simulink model "FM_Tut1"  (R2021a)
settings: Solver=VariableStepAuto  StartTime=0.0  StopTime=10.0  RelTol=1e-3
model workspace (MAT data in the model file):
  Ts = 4.16666666667e-06
  kf = 75000
libraries: dsparch4 x2, dspsnks4 x1, rtlsdr_book_library x1, dspstat3 x1, sdrrlib x1
settings Model: Creator=devan  LastModifiedBy=devan

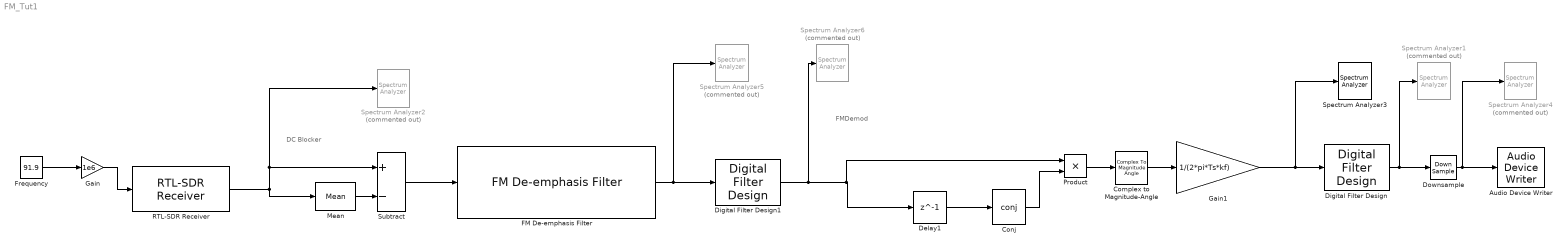
== system FM_Tut1 ==
  note: FMDemod
  note: DC Blocker
  Audio Device Writer : dspsnks4/Audio Device Writer  Driver=DirectSound  Device=Default  InheritSampleRate=on  SampleRate=44100  BitDepth=16-bit integer  BufferSize=4096  NumBuffers=10  DefaultOutputChannelMapping=on  OutputChannelMapping=1:2  OutputNumUnderrunSamples=off  DriverIdx=1  DeviceWarnFlag=''
  Complex to Magnitude-Angle : ComplexToMagnitudeAngle  Output=Angle
  Conj : Math  Operator=conj  SaturateOnIntegerOverflow=on
  Delay1 : Delay  DelayLength=1  InputProcessing=Columns as channels (frame based)
  Digital Filter Design : dsparch4/Digital Filter Design  mwdsp_browser_bugfix_var=off
  Digital Filter Design1 : dsparch4/Digital Filter Design  mwdsp_browser_bugfix_var=off
  Downsample : DownSample  N=5
  FM De-emphasis Filter : rtlsdr_book_library/FM Demod Tools/FM De-emphasis Filter  region=Europe, Asia  fs=240e3
      settings: SourceProductName=RTL-SDR Book Library
  Frequency : Constant  Value=91.9
  Gain : Gain  Gain=1e6
  Gain1 : Gain  Gain=1/(2*pi*Ts*kf)
  Mean : dspstat3/Mean  run=off  InputProcessing=Columns as channels (frame based)  reset_popup=None  directionMode=Each column  dimension=1  roiEnable=off  roiType=Rectangles  roiPortion=Entire ROI  roiOutput=Individual statistics for each ROI  roiFlag=off  roundingMode=Floor  overflowMode=off  outputDataTypeStr=Inherit: Same as accumulator  outputMin=[]  outputMax=[]  outputLastDataTypeStr=Inherit: Same as accumulator
  Product : Product
  RTL-SDR Receiver : sdrrlib/RTL-SDR Receiver  IPAddress=0  CenterFrequencySource=Input port  CenterFrequency=102.5e6  GainSource=Dialog  Gain=25  ADCRate=240e3  FrequencyCorrection=0  LostSamplesOutputPort=off  LatencyOutputPort=off  OutputDataType=single  FrameLength=1000  EnableBurstMode=off  NumFramesInBurst=20  sobjType=sdrr.internal.SDRRTLReceiverSL  dataUDPPort=-1  ctrlUDPPort=-1  subDeviceList=nosubdev  sdrBlockType=SDRBlockTypeSLT.SDRRxBlock  requester=UNUSED_BY_SFCN  sdrExecutionMode=SDRExecutionModeSLT.ExecModeHW  BypassUserLogic=off  DecimatorSelect=DDC decimator  SourceSelect=RF data  SineAmplitude=16000  EnableInternalClock=off  BypassIQBalance=off  IFBandwidth=40e6  ADCRateSource=Dialog  IntermediateFrequency=0  DecimationFactorSource=Dialog  DecimationFactor=512  RFFrequencyIsTunable=logical(1)  SampleTime=(1000)/(240e3)  IFBandwidthSource=Dialog  SineFrequency=30000  BypassDCBlockingFilter=off  IntermediateFrequencySource=Dialog  IQBalanceCoefficients=64  SkipAllHardwareResetAndInitialization=off  EnableIQCalibrationTable=on  CacheIQCalibrationTable=off  EnableOffsetTuning=off  EnableRTLAGC=off  EnableTestMode=off  EnableTunerAGC=off  FrequencyCorrectionSource=Dialog  NumMLBuffers=128  NumUSBBuffers=16  RTLCrystalFrequency=28800000  TunerCrystalFrequency=28800000
      settings: SourceProductBaseCode=RTLSDR
  Spectrum Analyzer{1..2,4..6} (5 alike) : SpectrumAnalyzer  Commented=on
  Spectrum Analyzer3 : SpectrumAnalyzer
  Subtract : Sum  Inputs=+-
  wires:
  Gain/1 -> RTL-SDR Receiver/1
  Frequency/1 -> Gain/1
  Subtract/1 -> FM De-emphasis Filter/1
  RTL-SDR Receiver/1 -> Spectrum Analyzer2/1, Subtract/1, Mean/1
  Mean/1 -> Subtract/2
  Digital Filter Design/1 -> Downsample/1, Spectrum Analyzer1/1
  Downsample/1 -> Audio Device Writer/1, Spectrum Analyzer4/1
  Gain1/1 -> Spectrum Analyzer3/1, Digital Filter Design/1
  Delay1/1 -> Conj/1
  Conj/1 -> Product/2
  FM De-emphasis Filter/1 -> Spectrum Analyzer5/1, Digital Filter Design1/1
  Complex to Magnitude-Angle/1 -> Gain1/1
  Product/1 -> Complex to Magnitude-Angle/1
  Digital Filter Design1/1 -> Spectrum Analyzer6/1, Product/1, Delay1/1
